simulink model "sum_tb"  (R2016b)
settings: Solver=VariableStepAuto  StartTime=0.0  StopTime=10.0  RelTol=1e-3
undefined symbols (not defined in the file or in its folder): A, N
libraries: xbsIndex_r4 x23, dspbuff3 x4, simulink x2, dspswit3 x2, JTAGRuntimeCosim_r4 x1
settings Model: Creator=root  LastModifiedBy=root

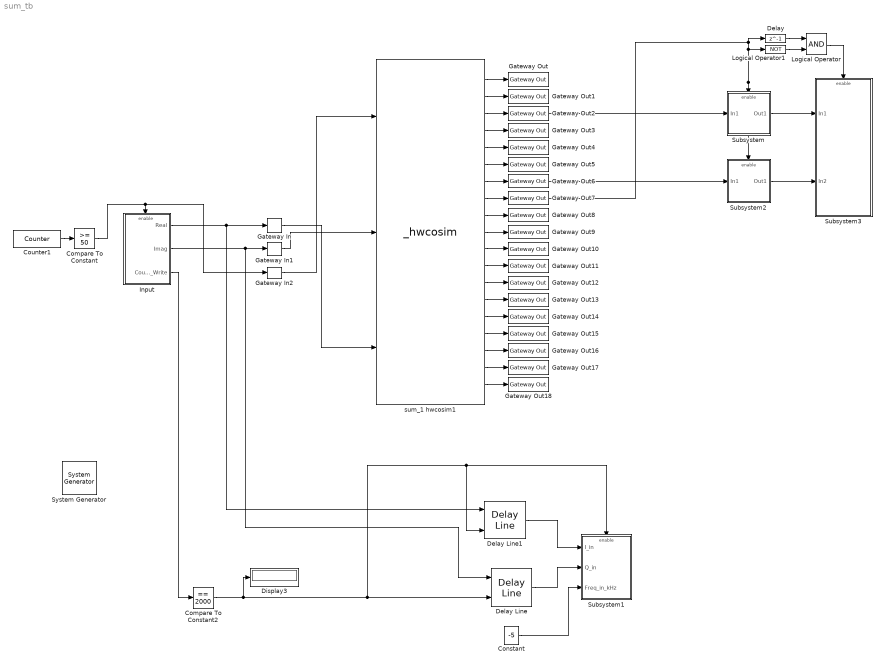
== system sum_tb ==
  " System Generator" : xbsIndex_r4/ System Generator  Tag=genX  xilinxfamily=virtex7  part=xc7vx485t  speed=-2  package=ffg1761  synthesis_tool=Vivado  clock_wrapper=Clock Enables  directory=./netlist  proj_type=Vivado  Synth_file=Vivado Synthesis Defaults  Impl_file=Vivado Implementation Defaults  testbench=off  simulink_period=1/(70e6)  sysclk_period=1000/70  dcm_input_clock_period=10  incr_netlist=off  trim_vbits=Everywhere in SubSystem  dbl_ovrd=According to Block Masks  core_generation=According to Block Masks  run_coregen=off  deprecated_control=off  eval_field=0  block_type=sysgen
  Compare To Constant : simulink/Logic and Bit Operations/Compare To Constant  relop=>=  const=50  OutDataTypeStr=boolean
  Compare To Constant2 : simulink/Logic and Bit Operations/Compare To Constant  relop===  const=2000  OutDataTypeStr=boolean
  Constant : Constant  Value=-5
  Counter1 : dspswit3/Counter  Direction=Up  CountEvent=Free running  CounterSize=16 bits  MaxCount=255  InitialCount=0  Output=Count  HitValue=32  ResetInput=off  SamplesPerFrame=1  Ts=1/(2e6)  CntDtype=uint16  HitDtype=Logical
  Delay : Delay  DelayLength=1
  Delay Line : dspbuff3/Delay Line  siz=2000  ic=0  directfeed=on  enable_output=on  hold_output=on  TreatMby1Signals=One channel  OutputFrames=off
  Delay Line1 : dspbuff3/Delay Line  siz=2000  ic=0  directfeed=on  enable_output=on  hold_output=on  TreatMby1Signals=One channel  OutputFrames=off
  Display3 : Display
      settings: Format=decimal (Stored Integer)
  Gateway In : xbsIndex_r4/Gateway In  gui_display_data_type=Fixed-point  arith_type="Signed  (2's comp)"  n_bits=12  bin_pt=0  preci_type=Single  exp_width=8  frac_width=24  rows=1  columns=1  quantization="Round  (unbiased: +/- Inf)"  overflow=Saturate  period=1/(70e6)  UseAsADC=off  ADCChannel='1'  interface=None  automatic_assignment=on  address_offset=hex2dec('00')  intf_name=''  intf_description=''  default_value=0  timing_constraint=None  locs_specified=off  LOCs={}  io_standard={}  inherit_from_input=off  hdl_port=on  dbl_ovrd=off  block_type=gatewayin
  Gateway In1 : xbsIndex_r4/Gateway In  gui_display_data_type=Fixed-point  arith_type="Signed  (2's comp)"  n_bits=12  bin_pt=0  preci_type=Single  exp_width=8  frac_width=24  rows=1  columns=1  quantization="Round  (unbiased: +/- Inf)"  overflow=Saturate  period=1/(70e6)  UseAsADC=off  ADCChannel='1'  interface=None  automatic_assignment=on  address_offset=hex2dec('00')  intf_name=''  intf_description=''  default_value=0  timing_constraint=None  locs_specified=off  LOCs={}  io_standard={}  inherit_from_input=off  hdl_port=on  dbl_ovrd=off  block_type=gatewayin
  Gateway In2 : xbsIndex_r4/Gateway In  gui_display_data_type=Boolean  arith_type=Boolean  n_bits=16  bin_pt=0  preci_type=Single  exp_width=8  frac_width=24  rows=1  columns=1  quantization="Round  (unbiased: +/- Inf)"  overflow=Saturate  period=1/(2e6)  UseAsADC=off  ADCChannel='1'  interface=None  automatic_assignment=on  address_offset=hex2dec('00')  intf_name=''  intf_description=''  default_value=0  timing_constraint=None  locs_specified=off  LOCs={}  io_standard={}  inherit_from_input=off  hdl_port=on  dbl_ovrd=off  block_type=gatewayin
  Gateway Out{,1..18} (19 alike) : xbsIndex_r4/Gateway Out  inherit_from_input=off  hdl_port=on  rows=1  columns=1  UseAsDAC=off  DACChannel='1'  interface=None  automatic_assignment=on  address_offset=hex2dec('00')  intf_name=''  intf_description=''  timing_constraint=None  locs_specified=off  LOCs={}  io_standard={}  block_type=gatewayout
  "Input " : Subsystem
  Logical Operator : Logic  AllPortsSameDT=off  OutDataTypeStr=boolean
  Logical Operator1 : Logic  Operator=NOT  AllPortsSameDT=off  OutDataTypeStr=boolean
  Subsystem : Subsystem
  Subsystem1 : Subsystem
  Subsystem2 : Subsystem
  Subsystem3 : Subsystem
  sum_1 hwcosim1 : JTAGRuntimeCosim_r4/_hwcosim  clkSrc=Single Stepped  hasCombinationalPath=on  bitfileName=/home/zaid/MTP/myrepo/sysgen/netlist/sum_1.bit  skipConfig=off  dispPartInfo=off  useZynqReconfigScript=on  cable=Auto Detect  speed=N/A  cablePort=N/A  cableLocation=Local  shareCable=off  design_xtable=|  engineDll=JTAGCosimEngine.dll  cableWaitTime=10  bscanPos=-1  IRLengths=[]  useWaitBox=1  hasBufgmux=on  Scheme=Cosim  useCmdProc=1  hasProc=0  useImpact=0  printLogFile=0  userChain=2  block_type=jtagcosim
      | {
      |     'clkWrapper' => 'sum_1',
      |     'burstMode' => false,
      |     'burstFifoDepth' => '1024',
      |     'shared_memories' => {},
      |     'clocksGcd' => 1,
      |     'device' => {
      |       'family' => 'virtex7',
      |       'part' => 'xc7vx485t',
      |       'package' => 'ffg1761',
      |       'speed' => '-2',
      |     },
      |     'ports' => {
      |       'gateway_in2' => {
      |         'direction' => 'in',
      |         'width' => 1,
      |         'name' => 'gateway_in2',
      |         'period' => 35,
      |         'icon_text' => 'Gateway In2',
      |         'type' => 'Bool',
      |         'arithmetic_type' => 'xlUnsigned',
      |         'dat_file' => 'sum_1_gateway_in2.dat',
      |         'bin_pt' => 0,
      |         'addr_offset' => 0,
      |         'bd_port_index' => 0,
      |       },
      |       'gateway_in1' => {
      |         'direction' => 'in',
      |         'width' => 12,
      |         'name' => 'gateway_in1',
      |         'period' => 1,
      |         'icon_text' => 'Gateway In1',
      |         'type' => 'Fix_12_0',
      |         'arithmetic_type' => 'xlSigned',
      |         'dat_file' => 'sum_1_gateway_in1.dat',
      |         'bin_pt' => 0,
      |         'addr_offset' => 4,
      |         'bd_port_index' => 1,
      |       },
      |       'gateway_in' => {
      |         'direction' => 'in',
      |         'width' => 12,
      |         'name' => 'gateway_in',
      |         'period' => 1,
      |         'icon_text' => 'Gateway In',
      |         'type' => 'Fix_12_0',
      |         'arithmetic_type' => 'xlSigned',
      |         'dat_file' => 'sum_1_gateway_in.dat',
      |         'bin_pt' => 0,
      |         'addr_offset' => 8,
      |         'bd_port_index' => 2,
      |       },
      |       'gateway_out' => {
      |         'direction' => 'out',
      |         'width' => 32,
      |         'name' => 'gateway_out',
      |         'period' => 1,
      |         'icon_text' => 'Gateway Out',
      |         'type' => 'UFix_32_0',
      |         'arithmetic_type' => 'xlUnsigned',
      |         'dat_file' => 'sum_1_gateway_out.dat',
      |         'bin_pt' => 0,
      |         'addr_offset' => 12,
      |         'bd_port_index' => 0,
      |       },
      |       'gateway_out2' => {
      |         'direction' => 'out',
      |         'width' => 1,
      |         'name' => 'gateway_out2',
      |         'period' => 1,
      |         'icon_text' => 'Gateway Out2',
      |         'type' => 'UFix_1_0',
      |         'arithmetic_type' => 'xlUnsigned',
      |         'dat_file' => 'sum_1_gateway_out2.dat',
      |         'bin_pt' => 0,
      |         'addr_offset' => 16,
      |         'bd_port_index' => 1,
      |       },
      |       'gateway_out3' => {
      |         'direction' => 'out',
      |         'width' => 25,
      |         'name' => 'gateway_out3',
      |         'period' => 1,
      |         'icon_text' => 'Gateway Out3',
      |         'type' => 'UFix_25_0',
      |         'arithmetic_type' => 'xlUnsigned',
      |         'dat_file' => 'sum_1_gateway_out3.dat',
      |         'bin_pt' => 0,
      |         'addr_offset' => 20,
      |         'bd_port_index' => 2,
      |       },
      |       'gateway_out1' => {
      |         'direction' => 'out',
      |         'width' => 1,
      |         'name' => 'gateway_out1',
      |         'period' => 1,
      |         'icon_text' => 'Gateway Out1',
      |         'type' => 'UFix_1_0',
      |         'arithmetic_type' => 'xlUnsigned',
      |         'dat_file' => 'sum_1_gateway_out1.dat',
      |         'bin_pt' => 0,
      |         'addr_offset' => 24,
      |         'bd_port_index' => 3,
      |       },
      |       'gateway_out16' => {
      |         'direction' => 'out',
      |         'width' => 10,
      |         'name' => 'gateway_out16',
      |         'period' => 1,
      |         'icon_text' => 'Gateway Out16',
      |         'type' => 'UFix_10_0',
      |         'arithmetic_type' => 'xlUnsigned',
      |         'dat_file' => 'sum_1_gateway_out16.dat',
      |         'bin_pt' => 0,
      |         'addr_offset' => 28,
      |         'bd_port_index' => 4,
      |       },
      |       'gateway_out17' => {
      |         'direction' => 'out',
      |         'width' => 4,
      |         'name' => 'gateway_out17',
      |         'period' => 1,
      |         'icon_text' => 'Gateway Out17',
      |         'type' => 'UFix_4_0',
      |         'arithmetic_type' => 'xlUnsigned',
      |         'dat_file' => 'sum_1_gateway_out17.dat',
      |         'bin_pt' => 0,
      |         'addr_offset' => 32,
      |         'bd_port_index' => 5,
      |       },
      |       'gateway_out4' => {
      |         'direction' => 'out',
      |         'width' => 25,
      |         'name' => 'gateway_out4',
      |         'period' => 1,
      |         'icon_text' => 'Gateway Out4',
      |         'type' => 'UFix_25_0',
      |         'arithmetic_type' => 'xlUnsigned',
      |         'dat_file' => 'sum_1_gateway_out4.dat',
      |         'bin_pt' => 0,
      |         'addr_offset' => 36,
      |         'bd_port_index' => 6,
      |       },
      |       'gateway_out5' => {
      |         'direction' => 'out',
      |         'width' => 1,
      |         'name' => 'gateway_out5',
      |         'period' => 1,
      |         'icon_text' => 'Gateway Out5',
      |         'type' => 'UFix_1_0',
      |         'arithmetic_type' => 'xlUnsigned',
      |         'dat_file' => 'sum_1_gateway_out5.dat',
      |         'bin_pt' => 0,
      |         'addr_offset' => 40,
      |         'bd_port_index' => 7,
      |       },
      |       'gateway_out6' => {
      |         'direction' => 'out',
      |         'width' => 9,
      |         'name' => 'gateway_out6',
      |         'period' => 1,
      |         'icon_text' => 'Gateway Out6',
      |         'type' => 'UFix_9_0',
      |         'arithmetic_type' => 'xlUnsigned',
      |         'dat_file' => 'sum_1_gateway_out6.dat',
      |         'bin_pt' => 0,
      |         'addr_offset' => 44,
      |         'bd_port_index' => 8,
      |       },
      |       'gateway_out7' => {
      |         'direction' => 'out',
      |         'width' => 9,
      |         'name' => 'gateway_out7',
      |         'period' => 1,
      |         'icon_text' => 'Gateway Out7',
      |         'type' => 'UFix_9_0',
      |         'arithmetic_type' => 'xlUnsigned',
      |         'dat_file' => 'sum_1_gateway_out7.dat',
      |         'bin_pt' => 0,
      |         'addr_offset' => 48,
      |         'bd_port_index' => 9,
      |       },
      |       'gateway_out18' => {
      |         'direction' => 'out',
      |         'width' => 32,
      |         'name' => 'gateway_out18',
      |         'period' => 1,
      |         'icon_text' => 'Gateway Out18',
      |         'type' => 'UFix_32_0',
      |         'arithmetic_type' => 'xlUnsigned',
      |         'dat_file' => 'sum_1_gateway_out18.dat',
      |         'bin_pt' => 0,
      |         'addr_offset' => 52,
      |         'bd_port_index' => 10,
      |       },
      |       'gateway_out8' => {
      |         'direction' => 'out',
      |         'width' => 3,
      |         'name' => 'gateway_out8',
      |         'period' => 1,
      |         'icon_text' => 'Gateway Out8',
      |         'type' => 'UFix_3_0',
      |         'arithmetic_type' => 'xlUnsigned',
      |         'dat_file' => 'sum_1_gateway_out8.dat',
      |         'bin_pt' => 0,
      |         'addr_offset' => 56,
      |         'bd_port_index' => 11,
      |       },
      |       'gateway_out9' => {
      |         'direction' => 'out',
      |         'width' => 1,
      |         'name' => 'gateway_out9',
      |         'period' => 1,
      |         'icon_text' => 'Gateway Out9',
      |         'type' => 'UFix_1_0',
      |         'arithmetic_type' => 'xlUnsigned',
      |         'dat_file' => 'sum_1_gateway_out9.dat',
      |         'bin_pt' => 0,
      |         'addr_offset' => 60,
      |         'bd_port_index' => 12,
      |       },
      |       'gateway_out10' => {
      |         'direction' => 'out',
      |         'width' => 8,
      |         'name' => 'gateway_out10',
      |         'period' => 1,
      |         'icon_text' => 'Gateway Out10',
      |         'type' => 'UFix_8_0',
      |         'arithmetic_type' => 'xlUnsigned',
      |         'dat_file' => 'sum_1_gateway_out10.dat',
      |         'bin_pt' => 0,
      |         'addr_offset' => 64,
      |         'bd_port_index' => 13,
      |       },
      |       'gateway_out11' => {
      |         'direction' => 'out',
      |         'width' => 100,
      |         'name' => 'gateway_out11',
      |         'period' => 1,
      |         'icon_text' => 'Gateway Out11',
      |         'type' => 'UFix_100_0',
      |         'arithmetic_type' => 'xlUnsigned',
      |         'dat_file' => 'sum_1_gateway_out11.dat',
      |         'bin_pt' => 0,
      |         'addr_offset' => 68,
      |         'bd_port_index' => 14,
      |       },
      |       'gateway_out12' => {
      |         'direction' => 'out',
      |         'width' => 100,
      |         'name' => 'gateway_out12',
      |         'period' => 1,
      |         'icon_text' => 'Gateway Out12',
      |         'type' => 'UFix_100_0',
      |         'arithmetic_type' => 'xlUnsigned',
      |         'dat_file' => 'sum_1_gateway_out12.dat',
      |         'bin_pt' => 0,
      |         'addr_offset' => 84,
      |         'bd_port_index' => 15,
      |       },
      |       'gateway_out13' => {
      |         'direction' => 'out',
      |         'width' => 4,
      |         'name' => 'gateway_out13',
      |         'period' => 1,
      |         'icon_text' => 'Gateway Out13',
      |         'type' => 'UFix_4_0',
      |         'arithmetic_type' => 'xlUnsigned',
      |         'dat_file' => 'sum_1_gateway_out13.dat',
      |         'bin_pt' => 0,
      |         'addr_offset' => 100,
      |         'bd_port_index' => 16,
      |       },
      |       'gateway_out14' => {
      |         'direction' => 'out',
      |         'width' => 25,
      |         'name' => 'gateway_out14',
      |         'period' => 1,
      |         'icon_text' => 'Gateway Out14',
      |         'type' => 'UFix_25_0',
      |         'arithmetic_type' => 'xlUnsigned',
      |         'dat_file' => 'sum_1_gateway_out14.dat',
      |         'bin_pt' => 0,
      |         'addr_offset' => 104,
      |         'bd_port_index' => 17,
      |       },
      |       'gateway_out15' => {
      |         'direction' => 'out',
      |         'width' => 10,
      |         'name' => 'gateway_out15',
      |         'period' => 1,
      |         'icon_text' => 'Gateway Out15',
      |         'type' => 'UFix_10_0',
      |         'arithmetic_type' => 'xlUnsigned',
      |         'dat_file' => 'sum_1_gateway_out15.dat',
      |         'bin_pt' => 0,
      |         'addr_offset' => 108,
      |         'bd_port_index' => 18,
      |       },
      |     },
      |   }
  wires:
  "Input "/1(Real) -> Delay Line1/1, Gateway In/1
  Counter1/1 -> Compare To Constant/1
  Compare To Constant/1 -> Gateway In2/1, "Input "/Enable
  Gateway In2/1 -> sum_1 hwcosim1/1
  Gateway In/1 -> sum_1 hwcosim1/3
  Gateway In1/1 -> sum_1 hwcosim1/2
  "Input "/3("Count_Write ") -> Compare To Constant2/1
  Delay Line/1 -> Subsystem1/2(Q_in)
  "Input "/2("Imag ") -> Delay Line/1, Gateway In1/1
  Compare To Constant2/1 -> Display3/1, Subsystem1/Enable, Delay Line1/2, Delay Line/2
  Delay Line1/1 -> Subsystem1/1(I_in)
  Constant/1 -> Subsystem1/3("Freq_in_kHz ")
  sum_1 hwcosim1/1 -> Gateway Out/1
  sum_1 hwcosim1/2 -> Gateway Out1/1
  sum_1 hwcosim1/3 -> Gateway Out2/1
  sum_1 hwcosim1/4 -> Gateway Out3/1
  sum_1 hwcosim1/5 -> Gateway Out4/1
  sum_1 hwcosim1/6 -> Gateway Out5/1
  sum_1 hwcosim1/7 -> Gateway Out6/1
  sum_1 hwcosim1/8 -> Gateway Out7/1
  sum_1 hwcosim1/9 -> Gateway Out8/1
  sum_1 hwcosim1/10 -> Gateway Out9/1
  sum_1 hwcosim1/11 -> Gateway Out10/1
  sum_1 hwcosim1/12 -> Gateway Out11/1
  sum_1 hwcosim1/13 -> Gateway Out12/1
  sum_1 hwcosim1/14 -> Gateway Out13/1
  sum_1 hwcosim1/15 -> Gateway Out14/1
  sum_1 hwcosim1/16 -> Gateway Out15/1
  sum_1 hwcosim1/17 -> Gateway Out16/1
  sum_1 hwcosim1/18 -> Gateway Out17/1
  sum_1 hwcosim1/19 -> Gateway Out18/1
  Gateway Out6/1 -> Subsystem2/1(In1)
  Gateway Out7/1 -> Delay/1, Subsystem2/Enable, Subsystem/Enable, Logical Operator1/1
  Gateway Out2/1 -> Subsystem/1(In1)
  Subsystem/1(Out1) -> Subsystem3/1(In1)
  Subsystem2/1(Out1) -> Subsystem3/2(In2)
  Delay/1 -> Logical Operator/1
  Logical Operator1/1 -> Logical Operator/2
  Logical Operator/1 -> Subsystem3/Enable

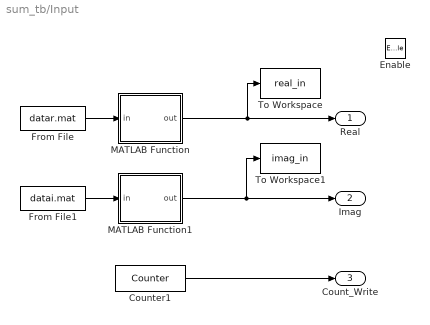
== system sum_tb/Input  ==
  Enable : EnablePort
  Counter1 : dspswit3/Counter  Direction=Up  CountEvent=Free running  CounterSize=User defined  MaxCount=2000  InitialCount=1  Output=Count  HitValue=32  ResetInput=off  SamplesPerFrame=1  Ts=1/(2e6)  CntDtype=uint16  HitDtype=Logical
  From File : FromFile  FileName=datar.mat  SampleTime=1/(2e6)
  From File1 : FromFile  FileName=datai.mat  SampleTime=1/(2e6)
  MATLAB Function : MATLAB Function  TreatAsAtomicUnit=on
  MATLAB Function1 : MATLAB Function  TreatAsAtomicUnit=on
  To Workspace : ToWorkspace  VariableName=real_in  SaveFormat=Timeseries  SampleTime=-1
  To Workspace1 : ToWorkspace  VariableName=imag_in  SaveFormat=Timeseries  SampleTime=-1
  Real : Outport
  "Imag " : Outport  Port=2
  "Count_Write " : Outport  Port=3
  wires:
  From File1/1 -> MATLAB Function1/1(in)
  MATLAB Function/1(out) -> To Workspace/1, Real/1
  From File/1 -> MATLAB Function/1(in)
  MATLAB Function1/1(out) -> To Workspace1/1, "Imag "/1
  Counter1/1 -> "Count_Write "/1

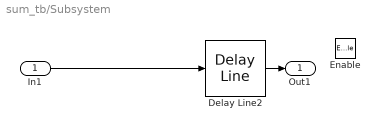
== system sum_tb/Subsystem ==
  In1 : Inport
  Enable : EnablePort
  Delay Line2 : dspbuff3/Delay Line  siz=2000  ic=0  directfeed=off  enable_output=off  hold_output=off  TreatMby1Signals=One channel  OutputFrames=off
  Out1 : Outport
  wires:
  Delay Line2/1 -> Out1/1
  In1/1 -> Delay Line2/1

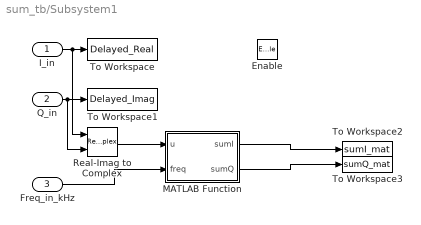
== system sum_tb/Subsystem1 ==
  I_in : Inport
  Q_in : Inport  Port=2
  "Freq_in_kHz " : Inport  Port=3
  Enable : EnablePort
  MATLAB Function : MATLAB Function  TreatAsAtomicUnit=on
  Real-Imag to Complex : RealImagToComplex
  To Workspace : ToWorkspace  VariableName=Delayed_Real  SaveFormat=Timeseries  SampleTime=-1
  To Workspace1 : ToWorkspace  VariableName=Delayed_Imag  SaveFormat=Timeseries  SampleTime=-1
  To Workspace2 : ToWorkspace  VariableName=sumI_mat  SaveFormat=Timeseries  SampleTime=-1
  To Workspace3 : ToWorkspace  VariableName=sumQ_mat  SaveFormat=Timeseries  SampleTime=-1
  wires:
  I_in/1 -> Real-Imag to Complex/1, To Workspace/1
  Q_in/1 -> Real-Imag to Complex/2, To Workspace1/1
  Real-Imag to Complex/1 -> MATLAB Function/1(u)
  "Freq_in_kHz "/1 -> MATLAB Function/2(freq)
  MATLAB Function/1(sumI) -> To Workspace2/1
  MATLAB Function/2(sumQ) -> To Workspace3/1

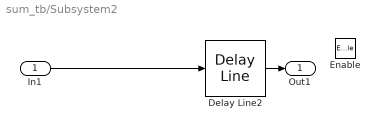
== system sum_tb/Subsystem2 ==
  In1 : Inport
  Enable : EnablePort
  Delay Line2 : dspbuff3/Delay Line  siz=2000  ic=0  directfeed=off  enable_output=off  hold_output=off  TreatMby1Signals=One channel  OutputFrames=off
  Out1 : Outport
  wires:
  Delay Line2/1 -> Out1/1
  In1/1 -> Delay Line2/1

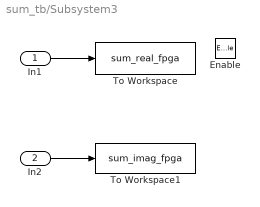
== system sum_tb/Subsystem3 ==
  In1 : Inport
  In2 : Inport  Port=2
  Enable : EnablePort
  To Workspace : ToWorkspace  VariableName=sum_real_fpga  SaveFormat=Timeseries  SampleTime=-1
  To Workspace1 : ToWorkspace  VariableName=sum_imag_fpga  SaveFormat=Timeseries  SampleTime=-1
  wires:
  In1/1 -> To Workspace/1
  In2/1 -> To Workspace1/1

== matlab function sum_tb/Input /MATLAB Function1 ==
  data: in input; out output
function out=toint(in)
in=in*2^16;
in=round(in);
out=fix(in);

== matlab function sum_tb/Input /MATLAB Function ==
  data: in input; out output
function out=toint(in)
in=in*2^16;
in=round(in);
out=fix(in);

== matlab function sum_tb/Subsystem1/MATLAB Function ==
  data: u input; freq input; sumI output; sumQ output
function [sumI,sumQ]=fcn(u,freq)
sample_time=1/(2e6);
time_axis=0:sample_time:sample_time*(length(u)-1);
carrier=exp(1i*2*pi*freq*time_axis*1e3);
y = u.*(carrier.');
y=fix(round(y*cordic_scale(16)));
code_out=goldcode(length(y),1);
sumI=zeros(1,length(y));sumQ=zeros(1,length(y));
for shft=1:length(code_out)
    codetemp=circshift(code_out',-shft);
    result=sum(codetemp.*y);
    sumI(shft)=real(result);
    sumQ(shft)=imag(result);
end
